simulink model "lab3_5_3"  (R2018a)
settings: Solver=VariableStepAuto  StartTime=0.0  StopTime=1500*Ts  RelTol=1e-3
values from neighbouring files (symbols this model uses):
  coefHybrid = [0 0.2 1 0.3 -0.4 -0.1 0.1 -0.05 -0.02 -0.01]    [lab3.m]
  Ts = 1    [lab3.m]
settings Model: Creator=leonardopedroso  LastModifiedBy=leonardopedroso

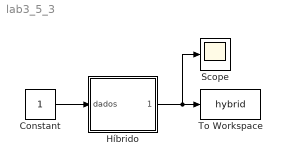
== system lab3_5_3 ==
  Constant : Constant
  Híbrido : Subsystem
  Scope : Scope
  To Workspace : ToWorkspace  VariableName=hybrid  SaveFormat=Timeseries  SampleTime=Ts/10
  wires:
  Constant/1 -> Híbrido/1(dados)
  Híbrido/1(híbrido) -> Scope/1, To Workspace/1

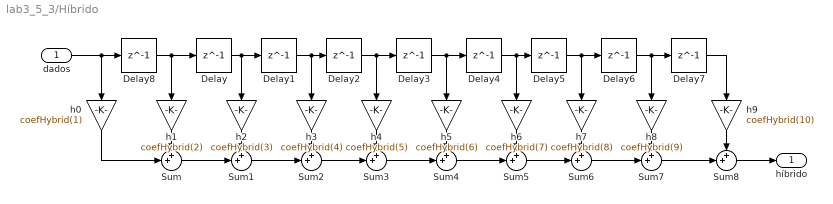
== system lab3_5_3/Híbrido ==
  dados : Inport
  Delay{,1..8} (9 alike) : Delay  DelayLength=1  SampleTime=Ts
  Sum{,1..8} (9 alike) : Sum  Inputs=++|
  h0 : Gain  Gain=coefHybrid(1)
  h1 : Gain  Gain=coefHybrid(2)
  h2 : Gain  Gain=coefHybrid(3)
  h3 : Gain  Gain=coefHybrid(4)
  h4 : Gain  Gain=coefHybrid(5)
  h5 : Gain  Gain=coefHybrid(6)
  h6 : Gain  Gain=coefHybrid(7)
  h7 : Gain  Gain=coefHybrid(8)
  h8 : Gain  Gain=coefHybrid(9)
  h9 : Gain  Gain=coefHybrid(10)
  híbrido : Outport
  wires:
  dados/1 -> h0/1, Delay8/1
  Delay/1 -> h2/1, Delay1/1
  Delay1/1 -> h3/1, Delay2/1
  Delay2/1 -> Delay3/1, h4/1
  Delay3/1 -> h5/1, Delay4/1
  Delay4/1 -> h6/1, Delay5/1
  Delay6/1 -> Delay7/1, h8/1
  Delay5/1 -> Delay6/1, h7/1
  Delay7/1 -> h9/1
  h0/1 -> Sum/2
  Delay8/1 -> h1/1, Delay/1
  h1/1 -> Sum/1
  Sum8/1 -> híbrido/1
  Sum/1 -> Sum1/2
  h2/1 -> Sum1/1
  h3/1 -> Sum2/1
  Sum1/1 -> Sum2/2
  h4/1 -> Sum3/1
  Sum2/1 -> Sum3/2
  h5/1 -> Sum4/1
  Sum3/1 -> Sum4/2
  h6/1 -> Sum5/1
  Sum4/1 -> Sum5/2
  Sum5/1 -> Sum6/2
  h7/1 -> Sum6/1
  h8/1 -> Sum7/1
  h9/1 -> Sum8/1
  Sum7/1 -> Sum8/2
  Sum6/1 -> Sum7/2
